simulink model "pil_main"  (R2020a)
settings: Solver=FixedStepDiscrete  StartTime=0.0  StopTime=inf  RelTol=1e-3
settings Model: SILPILModeSetting=veronly  SILPILSystemUnderTest=refmodels  Creator=asanchez  LastModifiedBy=asanchez
settings OptimizationCC: EnhancedBackFolding=on  PassReuseOutputArgsAs=Individual arguments  ZeroExternalMemoryAtStartup=off  ZeroInternalMemoryAtStartup=off  MaxStackSize=64  OptimizeBlockOrder=speed  DifferentSizesBufferReuse=on  OptimizationCustomize=off  EfficientTunableParamExpr=on
settings DebuggingCC: ParameterTunabilityLossMsg=error
settings HardwareCC: ProdBitPerPointer=32  ProdBitPerSizeT=32  ProdBitPerPtrDiffT=32  ProdLargestAtomicInteger=Long  ProdLargestAtomicFloat=Double  ProdWordSize=32  ProdHWDeviceType=ARM Compatible->ARM Cortex
settings SFSimCC: MATLABDynamicMemAlloc=off
settings RTWCC: SystemTargetFile=ert.tlc  HardwareBoard=Nuttx STM32H743ZI  TLCOptions="-aInlineSetEventsForThisBaseRateFcn=TLC_FALSE -aSuppressMultiTaskScheduler=TLC_FALSE     -aRateBasedStepFcn=1"  TemplateMakefile=ert_default_tmf  Toolchain=Nuttx Toolchain  CreateSILPILBlock=PIL  TargetLang=C++
settings CodeAppCC: ForceParamTrailComments=on  IgnoreCustomStorageClasses=off  OperatorAnnotations=on  SimulinkDataObjDesc=on  SFDataObjDesc=on  InsertBlockDesc=on
settings ERTTargetCC: TargetLangStandard=C++03 (ISO)  MultiInstanceERTCode=on  CodeInterfacePackaging=C++ class  RootIOFormat=Structure reference

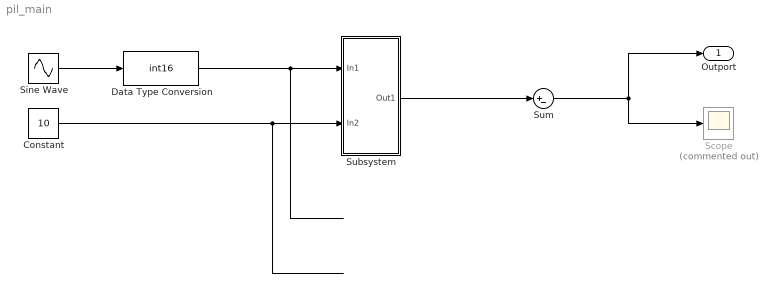
== system pil_main ==
  Constant : Constant  Value=10  OutDataTypeStr=int8  SampleTime=0.01
  Data Type Conversion : DataTypeConversion  OutDataTypeStr=int16
  Scope : Scope  Commented=on
  Sine Wave : Sin  SampleTime=0.01
  Subsystem : Subsystem  TreatAsAtomicUnit=on
  Sum : Sum  Inputs=|+-
  Outport : Outport
  wires:
  Subsystem/1(Out1) -> Sum/1
  Sum/1 -> Outport/1, Scope/1
  Constant/1 -> Subsystem/2(In2)
  Sine Wave/1 -> Data Type Conversion/1
  Data Type Conversion/1 -> Subsystem/1(In1)
  ? -> Sum/2

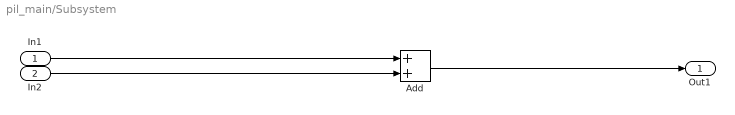
== system pil_main/Subsystem ==
  In1 : Inport
  In2 : Inport  Port=2
  Add : Sum
  Out1 : Outport
  wires:
  Add/1 -> Out1/1
  In2/1 -> Add/2
  In1/1 -> Add/1
